simulink model "FullModel"  (R2023a)
settings: Solver=VariableStepAuto  StartTime=0.0  StopTime=100  RelTol=1e-3
values from neighbouring files (symbols this model uses):
  SOC_LUT = [0.1 0.2 0.3 0.4 0.5 0.6 0.7 0.8 0.9 1]    [Final_Data.mat]
undefined symbols (not defined in the file or in its folder): B, D, I_P_TLU, Jd, Kcq, Kcs, Ld, Lq, m, n, n_, p, phi_mg, rho, Rs, t_iq, t_is, time
libraries: nesl_utility x4, fl_lib x3, spspowerguiLib x3, slpidlib x3, simulink x1, batteryecm_lib x1
settings Model: Creator=charu  LastModifiedBy=charu
settings DebuggingCC: AlgebraicLoopMsg=none

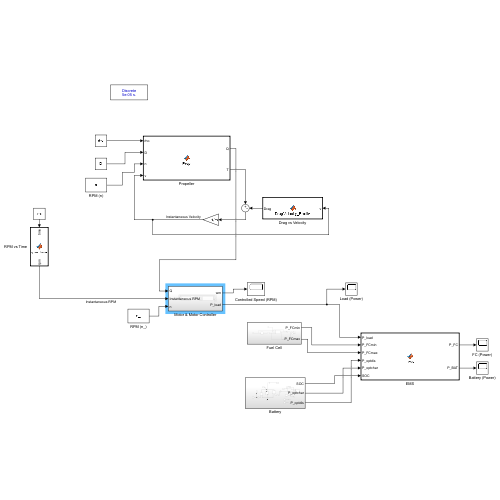
[thumbnail: Simulink's stored preview of the top-level diagram]
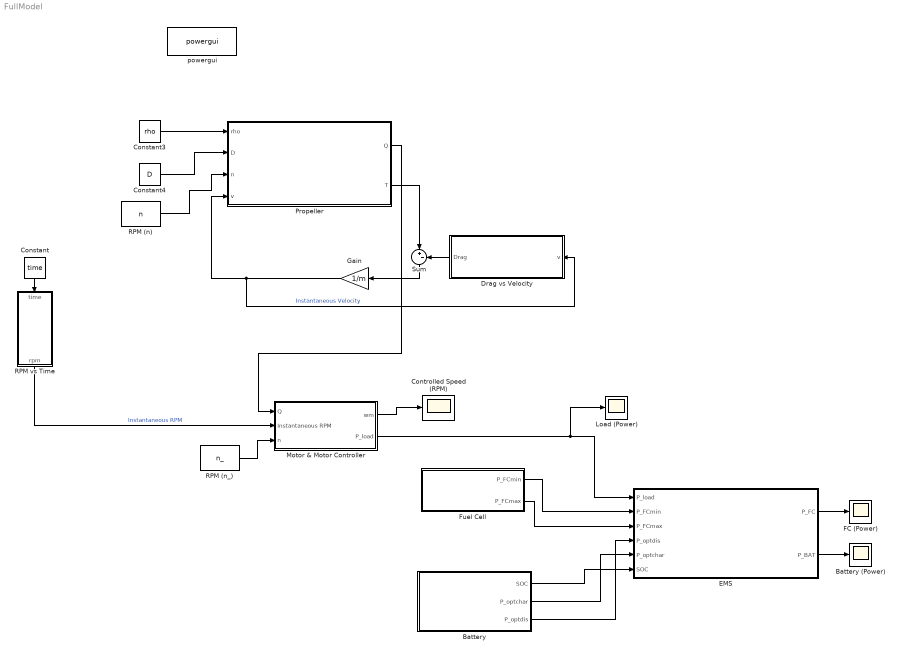
== system FullModel ==
  Battery : Subsystem
  Battery (Power) : Scope
  Constant : Constant  Value=time
  Constant3 : Constant  Value=rho
  Constant4 : Constant  Value=D
  Controlled Speed (RPM) : Scope
  Drag vs Velocity : MATLAB Function  TreatAsAtomicUnit=on
  EMS : MATLAB Function  TreatAsAtomicUnit=on
  FC (Power) : Scope
  Fuel Cell : Subsystem
  Gain : Gain  Gain=1/m
  Load (Power) : Scope
  Motor & Motor Controller : Subsystem
  Propeller : MATLAB Function  TreatAsAtomicUnit=on
  RPM (n) : Constant  Value=n
  RPM (n_) : Constant  Value=n_
  "RPM vs Time " : MATLAB Function  TreatAsAtomicUnit=on
  Sum : Sum  Inputs=|+-
  powergui : spspowerguiLib/powergui  Priority=1  SimulationMode=Discrete  SampleTime=50e-6  frequency=60  Iterations=50  frequencyindice=60  Pbase=100e6  ErrMax=1e-4  UnitsV=kV  UnitsW=MW  buscounter=0  FunctionMessages=off  echomessages=off  EnableUseOfTLC=off  CurrentSourceSwitches=off  DisableSnubberDevices=off  DisableRonSwitches=off  DisableVfSwitches=off  DisplayEquations=off  AutomaticDiscreteSolvers=off  SolverType=Tustin/Backward Euler (TBE)  Interpol=off  ExternalGateDelay=off  methode=off  Ts=100  x0status=blocks  SPID=on  SwTol=0  HookPort=off  NonlinearTolerance=1e-4  nMaxIteration=100  ContinueOnMaxIteration=off  RestoreLinks=warning  ResistiveCurrentMeasurement=off  Frange=[0:2:500]  Ylog=off  Xlog=on  ShowGrid=off  save=off  variable=ZData  structure=0  ZoomFFT=off  StartTime=0.0  cycles=1  DisplayStyle=1  fundamental=60  FreqAxis=off  MaxFrequency=1000  frequencyindicesteady=1  RmsSteady=1  display=off
  wires:
  Propeller/2(T) -> Sum/1
  Sum/1 -> Gain/1
  Gain/1 -> Drag vs Velocity/1(v), Propeller/4(v)  "Instantaneous Velocity"
  Constant/1 -> "RPM vs Time "/1(time)
  Constant3/1 -> Propeller/1(rho)
  Constant4/1 -> Propeller/2(D)
  RPM (n)/1 -> Propeller/3(n)
  Battery/1(SOC) -> EMS/6(SOC)
  Fuel Cell/1(P_FCmin) -> EMS/2(P_FCmin)
  Fuel Cell/2(P_FCmax) -> EMS/3(P_FCmax)
  Battery/2(P_optchar) -> EMS/5(P_optchar)
  Battery/3(P_optdis) -> EMS/4(P_optdis)
  Propeller/1(Q) -> Motor & Motor Controller/1(Q)
  Motor & Motor Controller/1(wm) -> Controlled Speed (RPM)/1
  Motor & Motor Controller/2(P_load) -> Load (Power)/1, EMS/1(P_load)
  Drag vs Velocity/1(Drag) -> Sum/2
  "RPM vs Time "/1(rpm) -> Motor & Motor Controller/2(Instantaneous RPM)  "Instantaneous RPM"
  RPM (n_)/1 -> Motor & Motor Controller/3(n)
  EMS/1(P_FC) -> FC (Power)/1
  EMS/2(P_BAT) -> Battery (Power)/1

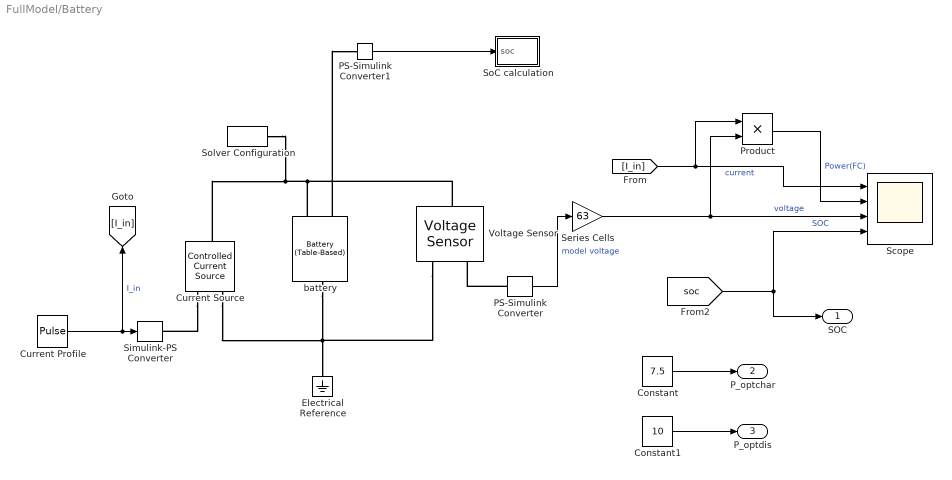
== system FullModel/Battery ==
  Constant : Constant  Value=7.5
  Constant1 : Constant  Value=10
  Current Source : fl_lib/Electrical/Electrical Sources/Controlled Current Source
  Current Profile : DiscretePulseGenerator  PulseType=Time based  Amplitude=-30  Period=20  PulseWidth=30  PhaseDelay=10
  Electrical Reference : fl_lib/Electrical/Electrical Elements/Electrical Reference
  PS-Simulink Converter : nesl_utility/PS-Simulink Converter  PhysicalDomain=network_engine_domain  SubClassName=ps_output  LeftPortType=input  RightPortType=output  PseudoPeriodic=off  Frequencies=[]  VectorFormat=1-D array  Unit=V  AffineConversion=off
  PS-Simulink Converter1 : nesl_utility/PS-Simulink Converter  PhysicalDomain=network_engine_domain  SubClassName=ps_output  LeftPortType=input  RightPortType=output  PseudoPeriodic=off  Frequencies=[]  VectorFormat=1-D array  Unit=inherit  AffineConversion=off
  Product : Product
  Scope : Scope  NumInputPorts=4
  Series Cells : Gain  Gain=63
  Simulink-PS Converter : nesl_utility/Simulink-PS Converter  PhysicalDomain=network_engine_domain  SubClassName=ps_input  LeftPortType=input  RightPortType=output  PseudoPeriodic=off  Frequencies=[]  NoiseDistribution=none  NoiseParameters=[]  Unit=A  AffineConversion=off  FilteringAndDerivatives=zero  SimscapeFilterOrder=1  InputFilterTimeConstant=.001  UdotUserProvided=0
  SoC calculation : Subsystem
  Solver Configuration : nesl_utility/Solver Configuration  PhysicalDomain=network_engine_domain  SubClassName=solver  LeftPortType=input  RightPortType=generic  Tones=[]  Harmonics=[]  SimulateNoise=off  Profile=off  UseLocalSampling=off  EnableSwitchedLinearOptims=on  FrequencyDomain=off  UseCCode=off  RelTol=0.001  AbsTol=1e-06  MinStep=1e-09  ToWorkspace=off  RevertToSquareIcSolve=off  NumHomotopyIterations=100  PhasorMode=off  PhasorModeNumHarmonics=1  ConsistencySolver=NEWTON_FTOL  IndexReductionMethod=DerivativeReplacement  DoDC=off  ResidualTolerance=1e-9  ConsistencyTolSource=GLOBAL  ConsistencyAbsTol=0.001  ConsistencyRelTol=0.001  ConsistencyTolFactor=0.001  UseLocalSolver=off  LocalSolverChoice=NE_BACKWARD_EULER_ADVANCER  ResolveIndetEquations=on  FunctionEvalNumThread=1  LocalSolverSampleTime=10  DoFixedCost=off  MaxNonlinIter=12  MaxModeIter=2  ComputeImpulses=off  ImpulseIterations=2  LinearAlgebra=Sparse  LinearAlgebraNumThread=0  EquationFormulation=NE_TIME_EF  DelaysMemoryBudget=1024  AutomaticFiltering=on  FilteringTimeConstant=0.001  PartitionStorageMethod=AS_NEEDED  PartitionMemoryBudget=1024  PartitionMethod=FAST
  Voltage Sensor : fl_lib/Electrical/Electrical Sensors/Voltage Sensor
  battery : batteryecm_lib/Battery (Table-Based)  SOC_vec=SOC_LUT  T_dependence=simscape.enum.tablebattery.temperature_dependence.no  prm_dir=simscape.enum.tablebattery.prm_dir.noCurrentDirectionality  T_vec=[273.15, 298.15, 323.15] K  V0_mat=[3.2, 3.1, 3.14; 3.25, 3.27, 3.3; 3.28, 3.31, 3.34; 3.33, 3.5, 3.59] V  V0_vec=Em V  V_range=[0, inf] V  R0_mat=[.03, .015, .002; .04, .017, .008; .039, .012, .006; .027, .013, .021] Ohm  R0_vec=R0 Ohm  R0_dis_mat=[.0117, .0085, .009; .011, .0085, .009; .0114, .0087, .0092; .0107, .0082, .0088; .0107, .0083, .0091; .0113, .0085, .0089; .0116, .0085, .0089] Ohm  R0_dis_vec=[.0085, .0085, .0087, .0082, .0083, .0085, .0085] Ohm  R0_ch_mat=[.0117, .0085, .009; .011, .0085, .009; .0114, .0087, .0092; .0107, .0082, .0088; .0107, .0083, .0091; .0113, .0085, .0089; .0116, .0085, .0089] Ohm  R0_ch_vec=[.0085, .0085, .0087, .0082, .0083, .0085, .0085] Ohm  AH=31 hr*A  prm_leak=simscape.enum.tablebattery.prm_leak.disabled  Rleak_vec=[8000, 7000, 6000] Ohm  Rleak=7e3 Ohm  extrapolation_option=simscape.enum.extrapolation.linear  SOC_port=simscape.enum.tablebattery.enable.yes  prm_dyn=2  R1_mat=[.089, .076, .01; .042, .022, .099; .019, .007, .002; .051, .043, .029] Ohm  R1_vec=R1 Ohm  tau1_mat=[44, 148, 235; 93, 110, 1000; 19, 27, 133; .5, 22, 3] s  tau1_vec=tau1 s  R2_mat=[.014, .382, .407; .028, .006, .007; .014, .007, .006; .333, .956, .912] Ohm  R2_vec=R2 Ohm  tau2_mat=[1, 44, 5644; 11, 24, 506; 2, 14, 330; 3310, 13419, 30216] s  tau2_vec=tau2 s  R3_mat=[.014, .382, .407; .028, .006, .007; .014, .007, .006; .333, .956, .912] Ohm  R3_vec=R3 Ohm  tau3_mat=[1, 44, 5644; 11, 24, 506; 2, 14, 330; 3310, 13419, 30216] s  tau3_vec=tau3 s  R4_mat=[.014, .382, .407; .028, .006, .007; .014, .007, .006; .333, .956, .912] Ohm  R4_vec=[.382, .006, .007, .956] Ohm  tau4_mat=[1, 44, 5644; 11, 24, 506; 2, 14, 330; 3310, 13419, 30216] s  tau4_vec=[44, 24, 14, 13419] s  R5_mat=[.014, .382, .407; .028, .006, .007; .014, .007, .006; .333, .956, .912] Ohm  R5_vec=[.382, .006, .007, .956] Ohm  tau5_mat=[1, 44, 5644; 11, 24, 506; 2, 14, 330; 3310, 13419, 30216] s  tau5_vec=[44, 24, 14, 13419] s  prm_fade=simscape.enum.tablebattery.prm_fade.equations  N0=100  dV0=0  dR0=0  dAH=0  dRleak=0  dR1=0  dR2=0  dR3=0  dR4=0  dR5=0  N0vec=[100, 200, 300]  Tfadevec=[298.15, 323.15] K  dV0vec=[0, 0, 0]  dR0vec=[0, 0, 0]  dAHvec=[0, 0, 0]  dRleakvec=[0, 0, 0]  dR1vec=[0, 0, 0]  dR2vec=[0, 0, 0]  dR3vec=[0, 0, 0]  dR4vec=[0, 0, 0]  dR5vec=[0, 0, 0]  dV0mat=[0, 0; 0, 0; 0, 0]  dR0mat=[0, 0; 0, 0; 0, 0]  dAHmat=[0, 0; 0, 0; 0, 0]  dRleakmat=[0, 0; 0, 0; 0, 0]  dR1mat=[0, 0; 0, 0; 0, 0]  dR2mat=[0, 0; 0, 0; 0, 0]  dR3mat=[0, 0; 0, 0; 0, 0]  dR4mat=[0, 0; 0, 0; 0, 0]  dR5mat=[0, 0; 0, 0; 0, 0]  prm_age_modeling=simscape.enum.tablebattery.prm_age_modeling.equation  storage_dt_age_vec=[0] d  storage_T_age_vec=[273] K  prm_age_OCV=simscape.enum.tablebattery.prm_age_OCV.OCV  OCV_age=0.9  SOC_age=0.6  prm_age_resistance=simscape.enum.tablebattery.prm_age.disabled  OCV_scaling_age_resistance=2.2134e6  OCV_offset_age_resistance=1.632e6  temp_exp_age_resistance=0.515833569 V  t_exp_age_resistance=0.75  T_age_vec_resistance=[273.15, 298.15, 323.15] K  dt_age_vec_resistance=[90, 180, 270, 360] d  dR0_age_vec=[0, 0, 0]  t_meas_dR0_age=100 d  dR0_age_mat=[0, 0, 0; 0, 0, 0; 0, 0, 0; 0, 0, 0]  prm_age_capacity=simscape.enum.tablebattery.prm_age.disabled  OCV_scaling_age_capacity=1.5097e07  OCV_offset_age_capacity=8.3625e06  temp_exp_age_capacity=0.6011 V  t_exp_age_capacity=0.75  T_age_vec_capacity=[273.15, 298.15, 323.15] K  dt_age_vec_capacity=[90, 180, 270, 360] d  dAH_age_vec=[0, 0, 0]  t_meas_dAH_age=100 d  dAH_age_mat=[0, 0, 0; 0, 0, 0; 0, 0, 0; 0, 0, 0]  thermal_port=simscape.enum.thermaleffects.omit  temperature=298.15 K  thermal_mass=30000 J/K  i_specify=off  i_priority=None  i=0 A  i_nominal_specify=off  i_nominal_unit=A  i_nominal_value=1  v_specify=off  v_priority=None  v=0 V  v_nominal_specify=off  v_nominal_unit=V  v_nominal_value=1  stateOfCharge_specify=on  stateOfCharge_priority=High  stateOfCharge=1  stateOfCharge_nominal_specify=off  stateOfCharge_nominal_unit=1  stateOfCharge_nominal_value=1  num_cycles_specify=off  num_cycles_priority=High  num_cycles=0  num_cycles_nominal_specify=off  num_cycles_nominal_unit=1  num_cycles_nominal_value=1  cell_temperature_specify=off  cell_temperature_priority=High  cell_temperature=298.15 K  cell_temperature_nominal_specify=off  cell_temperature_nominal_unit=K  cell_temperature_nominal_value=1
      settings: InternalSimscapePortConfiguration="{\"Bottom\":[],\"Left\":[{\"id\":\"p\",\"label\":\"+\",\"type\":\"foundation.electrical.electrical\"},{\"id\":\"soc\",\"label\":\"SOC\",\"type\":\"output\"}],\"Right\":[{\"id\":\"n\",\"label\":\"-\",\"type\":\"foundation.electrical.electrical\"}],\"Top\":[]}"
  SOC : Outport
  P_optchar : Outport  Port=2
  P_optdis : Outport  Port=3
  wires:
  Series Cells/1 -> Scope/3, Product/2  "voltage"
  [I_in] -> Product/1, Scope/1  "current"
  PS-Simulink Converter/1 -> Series Cells/1  "model voltage"
  PS-Simulink Converter1/1 -> SoC calculation/1(soc)
  Current Profile/1 -> Simulink-PS Converter/1, [I_in]  "I_in"
  [soc] -> SOC/1, Scope/4  "SOC"
  Product/1 -> Scope/2  "Power(FC)"
  Constant/1 -> P_optchar/1
  Constant1/1 -> P_optdis/1
  connections:
  battery/LConn1 -- Solver Configuration/RConn1 -- Current Source/LConn1 -- Voltage Sensor/LConn1
  battery/RConn1 -- Electrical Reference/LConn1 -- Current Source/RConn2 -- Voltage Sensor/RConn2
  battery/LConn2 -- PS-Simulink Converter1/LConn1
  PS-Simulink Converter/LConn1 -- Voltage Sensor/RConn1
  Current Source/RConn1 -- Simulink-PS Converter/RConn1

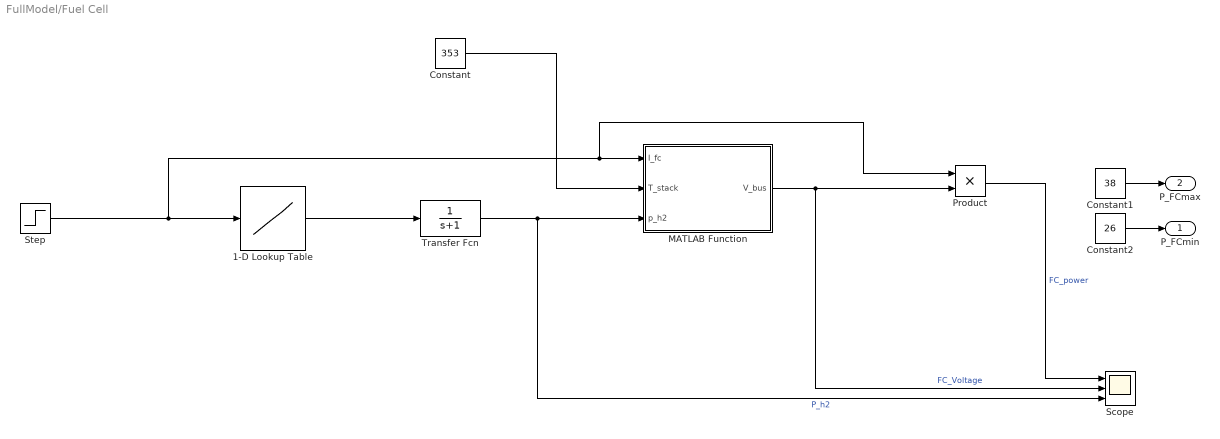
== system FullModel/Fuel Cell ==
  1-D Lookup Table : Lookup_n-D  NumberOfTableDimensions=1  BreakpointsForDimension1=I_P_TLU.Current  Table=I_P_TLU.Pressure  InternalRulePriority=Speed  RndMeth=Simplest
  Constant : Constant  Value=353
  Constant1 : Constant  Value=38
  Constant2 : Constant  Value=26
  MATLAB Function : MATLAB Function  TreatAsAtomicUnit=on
  Product : Product
  Scope : Scope  NumInputPorts=3
  Step : Step  Time=15  Before=107  After=154  SampleTime=0
  Transfer Fcn : TransferFcn  Denominator=[1 1]
  P_FCmin : Outport
  P_FCmax : Outport  Port=2
  wires:
  Transfer Fcn/1 -> Scope/3, MATLAB Function/3(p_h2)  "P_h2"
  MATLAB Function/1(V_bus) -> Scope/2, Product/2  "FC_Voltage"
  1-D Lookup Table/1 -> Transfer Fcn/1
  Product/1 -> Scope/1  "FC_power"
  Step/1 -> 1-D Lookup Table/1, Product/1, MATLAB Function/1(I_fc)
  Constant/1 -> MATLAB Function/2(T_stack)
  Constant2/1 -> P_FCmin/1
  Constant1/1 -> P_FCmax/1

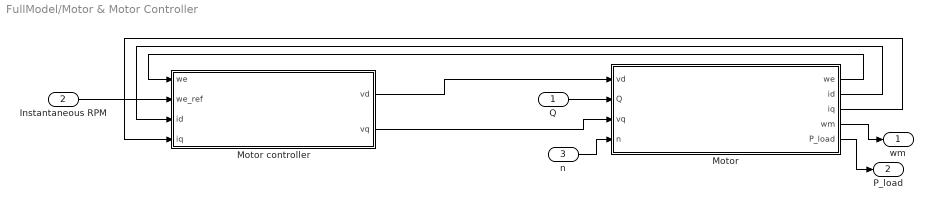
== system FullModel/Motor & Motor Controller ==
  Q : Inport
  Instantaneous RPM : Inport  Port=2
  n : Inport  Port=3
  Motor : Subsystem
  Motor controller : Subsystem
  wm : Outport
  P_load : Outport  Port=2
  wires:
  Motor/3(iq) -> Motor controller/4(iq)
  Motor/1(we) -> Motor controller/1(we)
  n/1 -> Motor/4(n)
  Q/1 -> Motor/2(Q)
  Motor controller/1(vd) -> Motor/1(vd)
  Instantaneous RPM/1 -> Motor controller/2(we_ref)
  Motor/2(id) -> Motor controller/3(id)
  Motor/5(P_load) -> P_load/1
  Motor/4(wm) -> wm/1
  Motor controller/2(vq) -> Motor/3(vq)

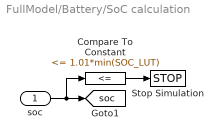
== system FullModel/Battery/SoC calculation ==
  soc : Inport
  Compare To Constant : simulink/Logic and Bit Operations/Compare To Constant  relop=<=  const=1.01*min(SOC_LUT)  OutDataTypeStr=boolean
  Stop Simulation : Stop
  tag scope: soc=global
  wires:
  soc/1 -> Compare To Constant/1, [soc]
  Compare To Constant/1 -> Stop Simulation/1

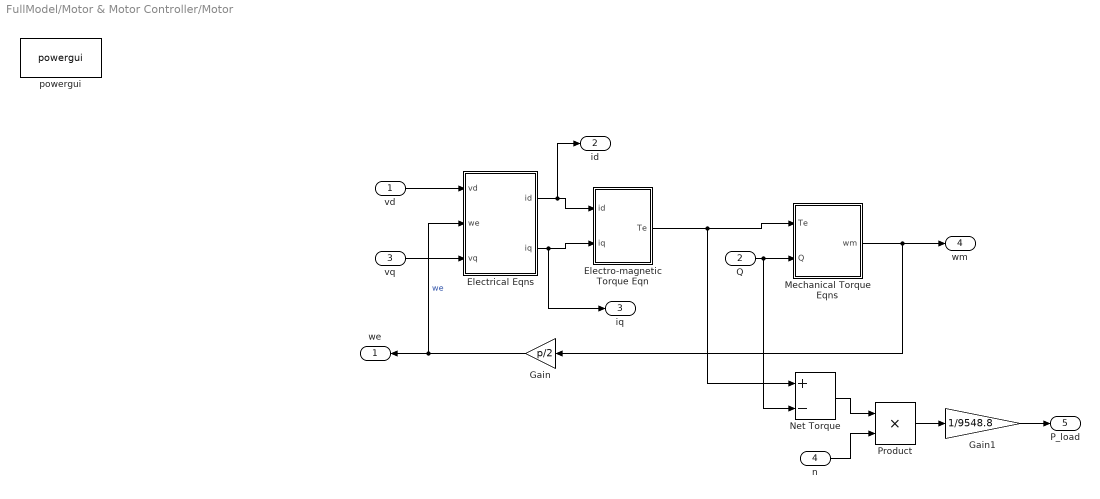
== system FullModel/Motor & Motor Controller/Motor ==
  vd : Inport
  Q : Inport  Port=2
  vq : Inport  Port=3
  n : Inport  Port=4
  Electrical Eqns : Subsystem
  Electro-magnetic Torque Eqn : Subsystem
  Gain : Gain  Gain=p/2
  Gain1 : Gain  Gain=1/9548.8
  Mechanical Torque Eqns : Subsystem
  Net Torque : Sum  Inputs=+-
  Product : Product
  powergui : spspowerguiLib/powergui  Priority=1  SimulationMode=Discrete  SampleTime=50e-6  frequency=60  Iterations=50  frequencyindice=60  Pbase=100e6  ErrMax=1e-4  UnitsV=kV  UnitsW=MW  buscounter=0  FunctionMessages=off  echomessages=off  EnableUseOfTLC=off  CurrentSourceSwitches=off  DisableSnubberDevices=off  DisableRonSwitches=off  DisableVfSwitches=off  DisplayEquations=off  AutomaticDiscreteSolvers=off  SolverType=Tustin/Backward Euler (TBE)  Interpol=off  ExternalGateDelay=off  methode=off  Ts=100  x0status=blocks  SPID=on  SwTol=0  HookPort=off  NonlinearTolerance=1e-4  nMaxIteration=100  ContinueOnMaxIteration=off  RestoreLinks=warning  ResistiveCurrentMeasurement=off  Frange=[0:2:500]  Ylog=off  Xlog=on  ShowGrid=off  save=off  variable=ZData  structure=0  ZoomFFT=off  StartTime=0.0  cycles=1  DisplayStyle=1  fundamental=60  FreqAxis=off  MaxFrequency=1000  frequencyindicesteady=1  RmsSteady=1  display=off
  we : Outport
  id : Outport  Port=2
  iq : Outport  Port=3
  wm : Outport  Port=4
  P_load : Outport  Port=5
  wires:
  Electrical Eqns/1(id) -> id/1, Electro-magnetic Torque Eqn/1(id)
  Gain/1 -> Electrical Eqns/2(we), we/1  "we"
  Electrical Eqns/2(iq) -> Electro-magnetic Torque Eqn/2(iq), iq/1
  Electro-magnetic Torque Eqn/1(Te) -> Net Torque/1, Mechanical Torque Eqns/1(Te)
  Mechanical Torque Eqns/1(wm) -> wm/1, Gain/1
  Q/1 -> Net Torque/2, Mechanical Torque Eqns/2(Q)
  vd/1 -> Electrical Eqns/1(vd)
  vq/1 -> Electrical Eqns/3(vq)
  Net Torque/1 -> Product/1
  n/1 -> Product/2
  Product/1 -> Gain1/1
  Gain1/1 -> P_load/1

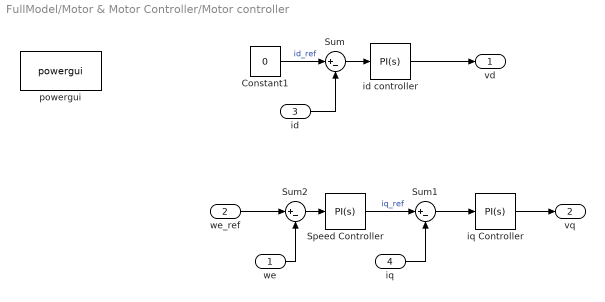
== system FullModel/Motor & Motor Controller/Motor controller ==
  we : Inport
  we_ref : Inport  Port=2
  id : Inport  Port=3
  iq : Inport  Port=4
  Constant1 : Constant  Value=0
  Speed Controller : slpidlib/PID Controller  Controller=PI  Form=Parallel  TimeDomain=Continuous-time  UseExternalTs=off  SampleTime=-1  IntegratorMethod=Forward Euler  FilterMethod=Forward Euler  ControllerParametersSource=internal  P=Kcs  I=Kcs/t_is  UseKiTs=off  D=0  N=100  UseFilter=on  TunerSelectOption=Transfer Function Based (PID Tuner App)  InitialConditionSource=internal  InitialConditionForIntegrator=0  InitialConditionForFilter=0  DifferentiatorICPrevScaledInput=0  ExternalReset=none  TrackingMode=off  Kt=1  LimitOutput=off  SatLimitsSource=internal  UpperSaturationLimit=inf  LowerSaturationLimit=-inf  LinearizeAsGain=on  AntiWindupMode=none  Kb=1  LimitIntegrator=off  UpperIntegratorSaturationLimit=inf  LowerIntegratorSaturationLimit=-inf  POutMin=[]  POutMax=[]  IOutMin=[]  IOutMax=[]  DOutMin=[]  DOutMax=[]  NOutMin=[]  NOutMax=[]  SumOutMin=[]  SumOutMax=[]  SaturationOutMin=[]  SaturationOutMax=[]  PParamMin=[]  PParamMax=[]  IParamMin=[]  IParamMax=[]  DParamMin=[]  DParamMax=[]  NParamMin=[]  NParamMax=[]  KbParamMin=[]  KbParamMax=[]  KtParamMin=[]  KtParamMax=[]  KbOutMin=[]  KbOutMax=[]  KtOutMin=[]  KtOutMax=[]  IntegratorOutMin=[]  IntegratorOutMax=[]  FilterOutMin=[]  FilterOutMax=[]  SumI1OutMin=[]  SumI1OutMax=[]  SumI2OutMin=[]  SumI2OutMax=[]  SumI3OutMin=[]  SumI3OutMax=[]  SumI4OutMin=[]  SumI4OutMax=[]  SumDOutMin=[]  SumDOutMax=[]  DifferentiatorOutMin=[]  DifferentiatorOutMax=[]  FilterDiffOutCoefMin=[]  FilterDiffOutCoefMax=[]  ReciprocalOutMin=[]  ReciprocalOutMax=[]  SumDenOutMin=[]  SumDenOutMax=[]  SumNumOutMin=[]  SumNumOutMax=[]  DivideOutMin=[]  DivideOutMax=[]  UdiffTsProdOutMin=[]  UdiffTsProdOutMax=[]  NTsProdOutMin=[]  NTsProdOutMax=[]  UintegralTsProdOutMin=[]  UintegralTsProdOutMax=[]  UngainTsProdOutMin=[]  UngainTsProdOutMax=[]  ClampingZeroOutDataTypeStr=Inherit: Inherit via back propagation  ClampingZeroOutMin=[]  ClampingZeroOutMax=[]  FilterDenConstantOutDataTypeStr=Inherit: Inherit via back propagation  FilterDenConstantOutMin=[]  FilterDenConstantOutMax=[]  PCopyOutDataTypeStr=Inherit: Inherit via back propagation  PCopyOutMin=[]  PCopyOutMax=[]  NCopyOutDataTypeStr=Inherit: Inherit via back propagation  NCopyOutMin=[]  NCopyOutMax=[]  IntegratorContinuousStateAttributes=''  IntegratorStateMustResolveToSignalObject=off  IntegratorRTWStateStorageClass=Auto  FilterContinuousStateAttributes=''  FilterStateMustResolveToSignalObject=off  FilterRTWStateStorageClass=Auto  ParallelPVariant=InternalParameters  IdealPVariant=Disabled  IVariant=InternalParameters  DVariant=Disabled  IntegratorVariant=Continuous  SatVariant=Disabled  AWVariant=Passthrough  PCopyVariant=Disabled  TRVariant=Disabled  FdbkBlocksVariant=Forward  IdealPFdbkVariant=Disabled  SatFdbkVariant=Disabled  DerivativeFilterVariant=Disabled  NVariant=Disabled  NCopyVariant=Disabled_SignalSpec  FilterICVariant=Disabled  IntegratorICVariant=InternalICs  ExternalResetVariant=Disabled  TRSumVariant=Passthrough  SumFdbkVariant=Disabled  SumVariant=Sum_PI  TsampFilterVariant=InternalTs  TsampNgainVariant=Passthrough  TsampIntegralVariant=Disabled_SignalSpec  ExternalSaturationOutDataTypeStr=Inherit: Same as second input
  Sum : Sum  Inputs=|+-
  Sum1 : Sum  Inputs=|+-
  Sum2 : Sum  Inputs=|+-
  id controller : slpidlib/PID Controller  Controller=PI  Form=Parallel  TimeDomain=Continuous-time  UseExternalTs=off  SampleTime=-1  IntegratorMethod=Forward Euler  FilterMethod=Forward Euler  ControllerParametersSource=internal  P=Kcq  I=Kcq/t_iq  UseKiTs=off  D=0  N=100  UseFilter=on  TunerSelectOption=Transfer Function Based (PID Tuner App)  InitialConditionSource=internal  InitialConditionForIntegrator=0  InitialConditionForFilter=0  DifferentiatorICPrevScaledInput=0  ExternalReset=none  TrackingMode=off  Kt=1  LimitOutput=off  SatLimitsSource=internal  UpperSaturationLimit=inf  LowerSaturationLimit=-inf  LinearizeAsGain=on  AntiWindupMode=none  Kb=1  LimitIntegrator=off  UpperIntegratorSaturationLimit=inf  LowerIntegratorSaturationLimit=-inf  POutMin=[]  POutMax=[]  IOutMin=[]  IOutMax=[]  DOutMin=[]  DOutMax=[]  NOutMin=[]  NOutMax=[]  SumOutMin=[]  SumOutMax=[]  SaturationOutMin=[]  SaturationOutMax=[]  PParamMin=[]  PParamMax=[]  IParamMin=[]  IParamMax=[]  DParamMin=[]  DParamMax=[]  NParamMin=[]  NParamMax=[]  KbParamMin=[]  KbParamMax=[]  KtParamMin=[]  KtParamMax=[]  KbOutMin=[]  KbOutMax=[]  KtOutMin=[]  KtOutMax=[]  IntegratorOutMin=[]  IntegratorOutMax=[]  FilterOutMin=[]  FilterOutMax=[]  SumI1OutMin=[]  SumI1OutMax=[]  SumI2OutMin=[]  SumI2OutMax=[]  SumI3OutMin=[]  SumI3OutMax=[]  SumI4OutMin=[]  SumI4OutMax=[]  SumDOutMin=[]  SumDOutMax=[]  DifferentiatorOutMin=[]  DifferentiatorOutMax=[]  FilterDiffOutCoefMin=[]  FilterDiffOutCoefMax=[]  ReciprocalOutMin=[]  ReciprocalOutMax=[]  SumDenOutMin=[]  SumDenOutMax=[]  SumNumOutMin=[]  SumNumOutMax=[]  DivideOutMin=[]  DivideOutMax=[]  UdiffTsProdOutMin=[]  UdiffTsProdOutMax=[]  NTsProdOutMin=[]  NTsProdOutMax=[]  UintegralTsProdOutMin=[]  UintegralTsProdOutMax=[]  UngainTsProdOutMin=[]  UngainTsProdOutMax=[]  ClampingZeroOutDataTypeStr=Inherit: Inherit via back propagation  ClampingZeroOutMin=[]  ClampingZeroOutMax=[]  FilterDenConstantOutDataTypeStr=Inherit: Inherit via back propagation  FilterDenConstantOutMin=[]  FilterDenConstantOutMax=[]  PCopyOutDataTypeStr=Inherit: Inherit via back propagation  PCopyOutMin=[]  PCopyOutMax=[]  NCopyOutDataTypeStr=Inherit: Inherit via back propagation  NCopyOutMin=[]  NCopyOutMax=[]  IntegratorContinuousStateAttributes=''  IntegratorStateMustResolveToSignalObject=off  IntegratorRTWStateStorageClass=Auto  FilterContinuousStateAttributes=''  FilterStateMustResolveToSignalObject=off  FilterRTWStateStorageClass=Auto  ParallelPVariant=InternalParameters  IdealPVariant=Disabled  IVariant=InternalParameters  DVariant=Disabled  IntegratorVariant=Continuous  SatVariant=Disabled  AWVariant=Passthrough  PCopyVariant=Disabled  TRVariant=Disabled  FdbkBlocksVariant=Forward  IdealPFdbkVariant=Disabled  SatFdbkVariant=Disabled  DerivativeFilterVariant=Disabled  NVariant=Disabled  NCopyVariant=Disabled_SignalSpec  FilterICVariant=Disabled  IntegratorICVariant=InternalICs  ExternalResetVariant=Disabled  TRSumVariant=Passthrough  SumFdbkVariant=Disabled  SumVariant=Sum_PI  TsampFilterVariant=InternalTs  TsampNgainVariant=Passthrough  TsampIntegralVariant=Disabled_SignalSpec  ExternalSaturationOutDataTypeStr=Inherit: Same as second input
  iq Controller : slpidlib/PID Controller  Controller=PI  Form=Parallel  TimeDomain=Continuous-time  UseExternalTs=off  SampleTime=-1  IntegratorMethod=Forward Euler  FilterMethod=Forward Euler  ControllerParametersSource=internal  P=Kcq  I=Kcq/t_iq  UseKiTs=off  D=0  N=100  UseFilter=on  TunerSelectOption=Transfer Function Based (PID Tuner App)  InitialConditionSource=internal  InitialConditionForIntegrator=0  InitialConditionForFilter=0  DifferentiatorICPrevScaledInput=0  ExternalReset=none  TrackingMode=off  Kt=1  LimitOutput=off  SatLimitsSource=internal  UpperSaturationLimit=inf  LowerSaturationLimit=-inf  LinearizeAsGain=on  AntiWindupMode=none  Kb=1  LimitIntegrator=off  UpperIntegratorSaturationLimit=inf  LowerIntegratorSaturationLimit=-inf  POutMin=[]  POutMax=[]  IOutMin=[]  IOutMax=[]  DOutMin=[]  DOutMax=[]  NOutMin=[]  NOutMax=[]  SumOutMin=[]  SumOutMax=[]  SaturationOutMin=[]  SaturationOutMax=[]  PParamMin=[]  PParamMax=[]  IParamMin=[]  IParamMax=[]  DParamMin=[]  DParamMax=[]  NParamMin=[]  NParamMax=[]  KbParamMin=[]  KbParamMax=[]  KtParamMin=[]  KtParamMax=[]  KbOutMin=[]  KbOutMax=[]  KtOutMin=[]  KtOutMax=[]  IntegratorOutMin=[]  IntegratorOutMax=[]  FilterOutMin=[]  FilterOutMax=[]  SumI1OutMin=[]  SumI1OutMax=[]  SumI2OutMin=[]  SumI2OutMax=[]  SumI3OutMin=[]  SumI3OutMax=[]  SumI4OutMin=[]  SumI4OutMax=[]  SumDOutMin=[]  SumDOutMax=[]  DifferentiatorOutMin=[]  DifferentiatorOutMax=[]  FilterDiffOutCoefMin=[]  FilterDiffOutCoefMax=[]  ReciprocalOutMin=[]  ReciprocalOutMax=[]  SumDenOutMin=[]  SumDenOutMax=[]  SumNumOutMin=[]  SumNumOutMax=[]  DivideOutMin=[]  DivideOutMax=[]  UdiffTsProdOutMin=[]  UdiffTsProdOutMax=[]  NTsProdOutMin=[]  NTsProdOutMax=[]  UintegralTsProdOutMin=[]  UintegralTsProdOutMax=[]  UngainTsProdOutMin=[]  UngainTsProdOutMax=[]  ClampingZeroOutDataTypeStr=Inherit: Inherit via back propagation  ClampingZeroOutMin=[]  ClampingZeroOutMax=[]  FilterDenConstantOutDataTypeStr=Inherit: Inherit via back propagation  FilterDenConstantOutMin=[]  FilterDenConstantOutMax=[]  PCopyOutDataTypeStr=Inherit: Inherit via back propagation  PCopyOutMin=[]  PCopyOutMax=[]  NCopyOutDataTypeStr=Inherit: Inherit via back propagation  NCopyOutMin=[]  NCopyOutMax=[]  IntegratorContinuousStateAttributes=''  IntegratorStateMustResolveToSignalObject=off  IntegratorRTWStateStorageClass=Auto  FilterContinuousStateAttributes=''  FilterStateMustResolveToSignalObject=off  FilterRTWStateStorageClass=Auto  ParallelPVariant=InternalParameters  IdealPVariant=Disabled  IVariant=InternalParameters  DVariant=Disabled  IntegratorVariant=Continuous  SatVariant=Disabled  AWVariant=Passthrough  PCopyVariant=Disabled  TRVariant=Disabled  FdbkBlocksVariant=Forward  IdealPFdbkVariant=Disabled  SatFdbkVariant=Disabled  DerivativeFilterVariant=Disabled  NVariant=Disabled  NCopyVariant=Disabled_SignalSpec  FilterICVariant=Disabled  IntegratorICVariant=InternalICs  ExternalResetVariant=Disabled  TRSumVariant=Passthrough  SumFdbkVariant=Disabled  SumVariant=Sum_PI  TsampFilterVariant=InternalTs  TsampNgainVariant=Passthrough  TsampIntegralVariant=Disabled_SignalSpec  ExternalSaturationOutDataTypeStr=Inherit: Same as second input
  powergui : spspowerguiLib/powergui  Priority=1  SimulationMode=Discrete  SampleTime=50e-6  frequency=60  Iterations=50  frequencyindice=60  Pbase=100e6  ErrMax=1e-4  UnitsV=kV  UnitsW=MW  buscounter=0  FunctionMessages=off  echomessages=off  EnableUseOfTLC=off  CurrentSourceSwitches=off  DisableSnubberDevices=off  DisableRonSwitches=off  DisableVfSwitches=off  DisplayEquations=off  AutomaticDiscreteSolvers=off  SolverType=Tustin/Backward Euler (TBE)  Interpol=off  ExternalGateDelay=off  methode=off  Ts=100  x0status=blocks  SPID=on  SwTol=0  HookPort=off  NonlinearTolerance=1e-4  nMaxIteration=100  ContinueOnMaxIteration=off  RestoreLinks=warning  ResistiveCurrentMeasurement=off  Frange=[0:2:500]  Ylog=off  Xlog=on  ShowGrid=off  save=off  variable=ZData  structure=0  ZoomFFT=off  StartTime=0.0  cycles=1  DisplayStyle=1  fundamental=60  FreqAxis=off  MaxFrequency=1000  frequencyindicesteady=1  RmsSteady=1  display=off
  vd : Outport
  vq : Outport  Port=2
  wires:
  Constant1/1 -> Sum/1  "id_ref"
  we_ref/1 -> Sum2/1
  Speed Controller/1 -> Sum1/1  "iq_ref"
  Sum2/1 -> Speed Controller/1
  Sum/1 -> id controller/1
  Sum1/1 -> iq Controller/1
  we/1 -> Sum2/2
  id controller/1 -> vd/1
  iq Controller/1 -> vq/1
  id/1 -> Sum/2
  iq/1 -> Sum1/2

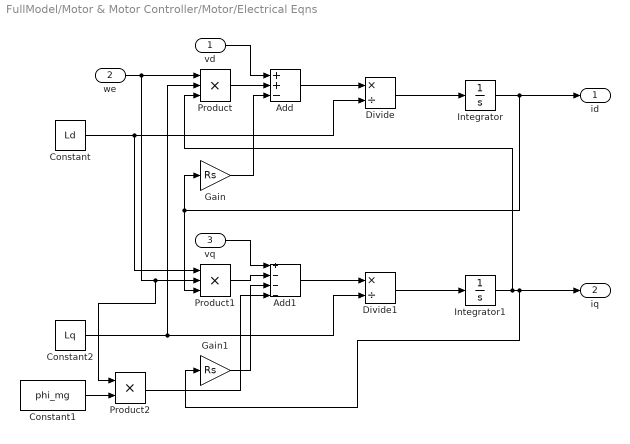
== system FullModel/Motor & Motor Controller/Motor/Electrical Eqns ==
  vd : Inport
  we : Inport  Port=2
  vq : Inport  Port=3
  Add : Sum  Inputs=++-
  Add1 : Sum  Inputs=+---
  Constant : Constant  Value=Ld
  Constant1 : Constant  Value=phi_mg
  Constant2 : Constant  Value=Lq
  Divide : Product  Inputs=*/
  Divide1 : Product  Inputs=*/
  Gain : Gain  Gain=Rs
  Gain1 : Gain  Gain=Rs
  Integrator : Integrator
  Integrator1 : Integrator
  Product : Product  Inputs=3
  Product1 : Product  Inputs=3
  Product2 : Product
  id : Outport
  iq : Outport  Port=2
  wires:
  Constant1/1 -> Product2/2
  Integrator/1 -> id/1, Product1/3, Gain/1
  Add/1 -> Divide/1
  Constant/1 -> Product1/1, Divide/2
  Product2/1 -> Add1/4
  Integrator1/1 -> iq/1, Gain1/1, Product/3
  vd/1 -> Add/1
  we/1 -> Product2/1, Product1/2, Product/1
  Constant2/1 -> Divide1/2, Product/2
  Divide/1 -> Integrator/1
  Product/1 -> Add/2
  Gain/1 -> Add/3
  Gain1/1 -> Add1/3
  Product1/1 -> Add1/2
  Add1/1 -> Divide1/1
  vq/1 -> Add1/1
  Divide1/1 -> Integrator1/1

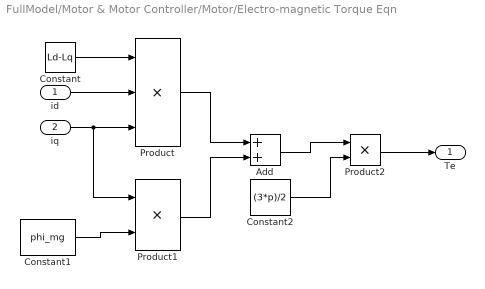
== system FullModel/Motor & Motor Controller/Motor/Electro-magnetic Torque Eqn ==
  id : Inport
  iq : Inport  Port=2
  Add : Sum
  Constant : Constant  Value=Ld-Lq
  Constant1 : Constant  Value=phi_mg
  Constant2 : Constant  Value=(3*p)/2
  Product : Product  Inputs=3
  Product1 : Product
  Product2 : Product
  Te : Outport
  wires:
  Constant2/1 -> Product2/2
  Product1/1 -> Add/2
  id/1 -> Product/2
  Constant1/1 -> Product1/2
  iq/1 -> Product1/1, Product/3
  Product/1 -> Add/1
  Constant/1 -> Product/1
  Add/1 -> Product2/1
  Product2/1 -> Te/1

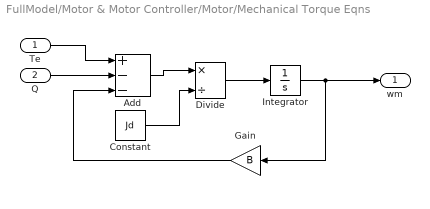
== system FullModel/Motor & Motor Controller/Motor/Mechanical Torque Eqns ==
  Te : Inport
  Q : Inport  Port=2
  Add : Sum  Inputs=+--
  Constant : Constant  Value=Jd
  Divide : Product  Inputs=*/
  Gain : Gain  Gain=B
  Integrator : Integrator
  wm : Outport
  wires:
  Constant/1 -> Divide/2
  Integrator/1 -> Gain/1, wm/1
  Divide/1 -> Integrator/1
  Te/1 -> Add/1
  Add/1 -> Divide/1
  Gain/1 -> Add/3
  Q/1 -> Add/2

== matlab function FullModel/EMS ==
  data: P_load input; P_FCmin input; P_FCmax input; P_optdis input; P_optchar input; SOC input; P_FC output; P_BAT output
function [P_FC,P_BAT] = EMS(P_load,P_FCmin,P_FCmax,P_optdis,P_optchar,SOC)
    num = length(P_load);  
    P_FC = zeros(num, 1);  
    P_BAT = zeros(num, 1); 
    for i = 1:num
        if SOC > 0.8 
            if P_load(i) <= P_FCmin
                P_FC(i) = P_FCmin;
                P_BAT(i) = P_FCmin - P_load(i);
            elseif P_load(i) > P_FCmin && P_load(i) <= P_FCmin + P_optdis 
                P_FC(i) = P_FCmin;
                P_BAT(i) = P_load(i) - P_FCmin;
            elseif P_load(i) > P_optdis + P_FCmax && P_load(i) <= P_FCmax + P_optdis
                P_FC(i) = P_load(i) - P_optdis;
                P_BAT(i) = P_optdis;
            elseif P_load(i) > P_optdis + P_FCmax
                P_FC(i) = P_FCmax;
                P_BAT(i) = P_load(i) - P_FCmax;
            end
        elseif SOC >= 0.5 && SOC <= 0.8
            if P_load(i) <= P_FCmin
                P_FC(i) = P_FCmin;
                P_BAT(i) = P_FCmin - P_load(i);
            end
        elseif SOC < 0.5
            if P_load(i) > P_FCmax
                P_FC(i) = P_FCmax;
                P_BAT(i) = P_load(i) - P_FCmax;
            elseif P_load(i) <= P_FCmax - P_optchar
                P_FC(i) = P_load(i);
                P_BAT(i) = 0;
            elseif P_load(i) > P_FCmax - P_optchar
                P_FC(i) = P_FCmax;
                P_BAT(i) = P_FCmax - P_load(i);
            end
        end
    end
end

== matlab function FullModel/Propeller ==
  data: Q output; rho input; D input; n input; v input; T output
function [Q,T] = Prop(rho,D,n,v)
% Ae/Ao = 1.050 ,No.of blades = 3 and P/D = 1.4 
    J_Q = [
    0
    0.035633656
    0.080186344
    0.11803914
    0.151453656
    0.18931707
    0.233837905
    0.280588497
    0.318451911
    0.358534465
    0.391948981
    0.429780541
    0.467633338
    0.507694656
    0.545547452
    0.585619388
    0.630140223
    0.670222777
    0.712513853
    0.743666757
    0.77704942
    0.832665954
    0.883833591
    0.92833319
    0.972790316
    1.021685724
    1.077217315
    1.121600117
    1.168148969
    1.210238305
    1.245564042
    1.276440882
    1.294013498
    1.315981923
    1.331303546
    1.342186888
    1.355268135
    1.363932337
    1.374794444
    1.381207653
    1.392037906
    1.398451115
    1.402634565
    1.406934813
];

    KQ_ = [0
0.028708134
0.066985646
0.09569378
0.124401914
0.155502392
0.186602871
0.220095694
0.251196172
0.282296651
0.311004785
0.33492823
0.363636364
0.389952153
0.418660287
0.447368421
0.4784689
0.509569378
0.538277512
0.557416268
0.578947368
0.610047847
0.638755981
0.66507177
0.681818182
0.698564593
0.710526316
0.710526316
0.698564593
0.681818182
0.641148325
0.598086124
0.557416268
0.507177033
0.459330144
0.411483254
0.358851675
0.311004785
0.258373206
0.203349282
0.14354067
0.088516746
0.031100478
0];

    J_T = [0
0.030133586
0.063314509
0.114248552
0.16298469
0.196197466
0.229378389
0.267029445
0.311327303
0.351165646
0.388784848
0.417559344
0.457387069
0.488380705
0.523812621
0.556993543
0.587976561
0.621178719
0.656589399
0.694208602
0.727389524
0.760612918
0.787147038
0.820349196
0.860187539
0.897806741
0.931008899
0.964200439
0.997402597
1.03280266
1.070421862
1.103634638
1.141275076
1.181113419
1.214326195
1.247528353
1.280741129
1.313943287
1.347145445
1.380358221
1.402496533
];

    KT_ = [0.796650718
0.789473684
0.765550239
0.741626794
0.722488038
0.705741627
0.681818182
0.66507177
0.645933014
0.622009569
0.598086124
0.581339713
0.555023923
0.538277512
0.5215311
0.497607656
0.4784689
0.459330144
0.437799043
0.413875598
0.389952153
0.375598086
0.354066986
0.33492823
0.311004785
0.28708134
0.267942584
0.246411483
0.227272727
0.203349282
0.179425837
0.162679426
0.14354067
0.119617225
0.102870813
0.083732057
0.066985646
0.04784689
0.028708134
0.011961722
0
];
    for i = length(n)
        J = v/(n(i)*D);
        KQ_fit = polyfit(J_Q,KQ_,2); 
        KT_fit = polyfit(J_T,KT_,1);
        KQ = polyval(KQ_fit, J);
        KT = polyval(KT_fit, J);
        T = KT * rho * n(i)^2 * D^4;
        Q = KQ * rho * n(i)^2 * D^5;
    end
end

== matlab function FullModel/Fuel Cell/MATLAB Function ==
  data: I_fc input; T_stack input; p_h2 input; V_bus output
function V_bus = fcn(I_fc,T_stack,p_h2)                %T_stack in K, T_fc in A, V_bus in V
    F = 96485.33;       
    R = 8.31447;
    i_lim = 1.4;
    A_cell = 500;
    N_cell = 300;

    E_cell = -237.14e+3/(-2*F);
    i_cell = I_fc/A_cell;
    
    i0 = 8e-05;
    alpha = 0.5;
    t_membrane = 125e-4;
    
    a = 0.5;
    lambda_m = 0.043 + 17.81*a - 39.85*a^2 + 36*a^3;
    sigma_30 = 0.005139*lambda_m - 0.00326;
    sigma = sigma_30*exp(1268*(1/303.15 - 1/T_stack));
    
    b = (R*T_stack)/(2*alpha*F);  

    V_nernst = E_cell + R*T_stack/(2*F) * log((3/4)^(1/2)*p_h2^(3/2));

    V_act = b*log(i_cell/i0);

    R_ohm = t_membrane/sigma;
    V_ohm = i_cell*R_ohm;

    V_conc = -R*T_stack/(2*F) * log(1-(i_cell/i_lim));          
    V_cell = V_nernst - V_act - V_ohm - V_conc;


    V_bus = V_cell*N_cell;
end

== matlab function FullModel/Drag vs Velocity ==
  data: v input; Drag output
function Drag = DragVelocity_Profile(v)
    Drag_ = [0
2.40165157
3.164117316
3.385663625
3.683299572
1.921181996
1.667962675
1.568170036
1.832926016
1.978032659
2.280974598];
    v_ = [0
4.545454545
9.090909091
13.63636364
16.898989
17.2020202
22.72727273
27.27272727
31.81818182
36.36363636
40.90909091];
    D_vfit = polyfit(v_,Drag_,1); 
    Drag = polyval(D_vfit, v);
end

== matlab function FullModel/RPM vs Time  ==
  data: time input; rpm output
function rpm = rpm_time(time)
    time_ = [0
1.6
3.2
4.8
6.4
8
9.6
11.2
12.8
14.4
16
17.6
19.2
20.8
22.4
24
25.6
27.2
28.8
30.4
32
33.6
35.2
36.8
38.4
40
41.6
43.2
44.8
46.4
48
49.6
51.2
52.8
54.4
56
57.6
59.2
60.8
62.4
64
65.6
67.2
68.8
70.4
72
73.6
75.2
76.8
78.4
80
81.6
83.2
84.8
86.4
88
89.6
91.2
92.8
94.4
96
97.6];
    rpm_ = [0
500
500
500
500
1000
2000
3000
4000
3000
3000
3000
3000
3300
3300
3300
3000
3000
3000
3000
3000
3500
3500
3500
3500
3000
3000
3000
2500
2000
0
0
500
1000
2000
3000
4000
3000
3000
3000
3000
3300
3300
3300
3000
3000
3000
3000
3000
3500
3500
3500
3500
3000
3000
3000
3000
3000
3000
2500
2000
0];
    rpm_time = polyfit(time_,rpm_,1);
    rpm = zeros(size(time_));
    for i = 1:length(time)
        rpm(i) = polyval(rpm_time, time(i));
    end
end
